simulink model "Distribution_v2"  (Simulink 7.9)
settings: Solver=VariableStepDiscrete  StartTime=0.0  StopTime=1000  RelTol=1e-3
libraries: simeventslib x35
(part 3 of 6)

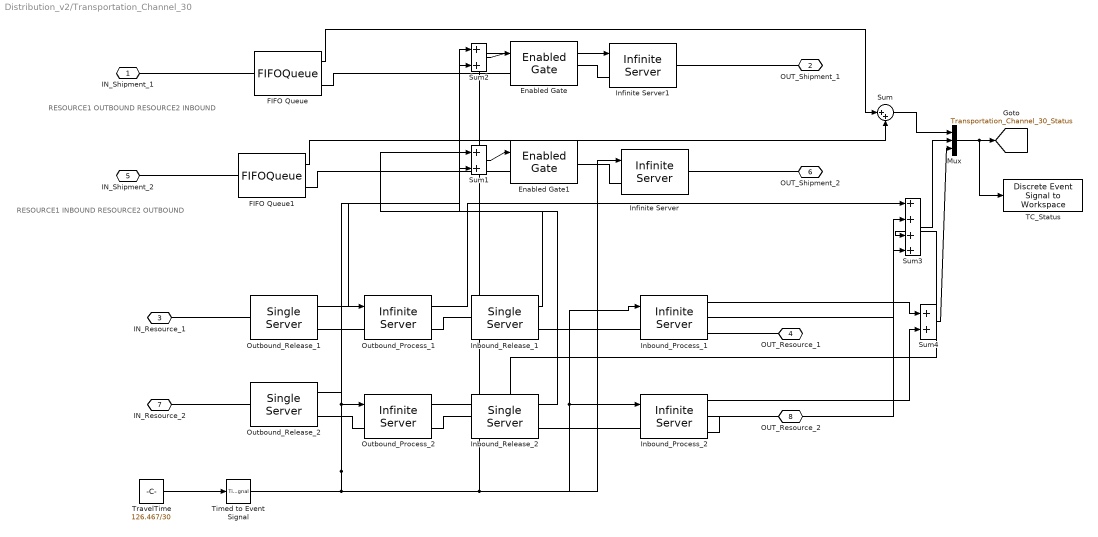
== system Distribution_v2/Transportation_Channel_30 ==
  note: RESOURCE1 OUTBOUND
      | RESOURCE2 INBOUND
  note: RESOURCE1 INBOUND
      | RESOURCE2 OUTBOUND
  Enabled Gate : EnabledGate
  Enabled Gate1 : EnabledGate
  FIFO Queue : FIFOQueue  Capacity=inf  StatNumberInBlock=on
      settings: OutputPortMap=o1
  FIFO Queue1 : FIFOQueue  Capacity=inf  StatNumberInBlock=on
      settings: OutputPortMap=o1
  Inbound_Process_1 : InfiniteServer  ServiceTimeFrom=Signal port t  ServiceTime=(76.7)/30  StatNumberDeparted=on  StatNumberInBlock=on
      settings: OutputPortMap=o0,o1
  Inbound_Process_2 : InfiniteServer  ServiceTimeFrom=Signal port t  ServiceTime=(76.7)/30  StatNumberDeparted=on  StatNumberInBlock=on
      settings: OutputPortMap=o0,o1
  Inbound_Release_1 : SingleServer  ServiceTime=0  StatNumberInBlock=on
      settings: OutputPortMap=o1
  Inbound_Release_2 : SingleServer  ServiceTime=0  StatNumberInBlock=on
      settings: OutputPortMap=o1
  Infinite Server : InfiniteServer  ServiceTimeFrom=Signal port t  ServiceTime=(76.7)/30
  Infinite Server1 : InfiniteServer  ServiceTimeFrom=Signal port t  ServiceTime=(76.7)/30
  Mux : Mux  Inputs=3
  Outbound_Process_1 : InfiniteServer  ServiceTimeFrom=Signal port t  ServiceTime=(76.7)/30  StatNumberInBlock=on
      settings: OutputPortMap=o1
  Outbound_Process_2 : InfiniteServer  ServiceTimeFrom=Signal port t  ServiceTime=(76.7)/30  StatNumberInBlock=on
      settings: OutputPortMap=o1
  Outbound_Release_1 : SingleServer  ServiceTime=0  StatNumberInBlock=on
      settings: OutputPortMap=o1
  Outbound_Release_2 : SingleServer  ServiceTime=0  StatNumberInBlock=on
      settings: OutputPortMap=o1
  Sum{,1..2,4} (4 alike) : Sum  Inputs=|++
  Sum3 : Sum  Inputs=|++++
  TC_Status : simeventslib/SimEvents Sinks/Discrete Event Signal to Workspace  VariableName=Transportation_Channel_30_Status  SaveFormat=Structure With Time  isMonitorOnly=off  isRecordIC=off
  Timed to Event Signal : TimedToEventSignal
  TravelTime : Constant  Value=126.467/30
  IN_Shipment_1 : PMIOPort  Port=1  Side=Left
  OUT_Shipment_1 : PMIOPort  Port=2  Side=Right
  IN_Resource_1 : PMIOPort  Port=3  Side=Left
  OUT_Resource_1 : PMIOPort  Port=4  Side=Right
  IN_Shipment_2 : PMIOPort  Port=5  Side=Left
  OUT_Shipment_2 : PMIOPort  Port=6  Side=Right
  IN_Resource_2 : PMIOPort  Port=7  Side=Left
  OUT_Resource_2 : PMIOPort  Port=8  Side=Right
  tag scope: Transportation_Channel_30_Status=global
  wires:
  Sum4/1 -> Mux/3
  Inbound_Process_2/1 -> Sum4/2
  Inbound_Process_1/1 -> Sum4/1
  Inbound_Process_2/2 -> Sum3/4
  Outbound_Process_2/1 -> Sum3/3
  Inbound_Process_1/2 -> Sum3/2
  Outbound_Process_1/1 -> Sum3/1
  Sum3/1 -> Mux/2
  Sum/1 -> Mux/1
  Mux/1 -> TC_Status/1, [Transportation_Channel_30_Status]
  Inbound_Release_2/1 -> Sum2/2
  Outbound_Release_1/1 -> Sum2/1
  Sum2/1 -> Enabled Gate/1
  Inbound_Release_1/1 -> Sum1/1
  Outbound_Release_2/1 -> Sum1/2
  Sum1/1 -> Enabled Gate1/1
  Timed to Event Signal/1 -> Infinite Server/1, Inbound_Process_2/1, Inbound_Process_1/1, Infinite Server1/1, Outbound_Process_2/1, Outbound_Process_1/1
  TravelTime/1 -> Timed to Event Signal/1
  FIFO Queue/1 -> Sum/1
  FIFO Queue1/1 -> Sum/2
  connections:
  Inbound_Process_1/RConn1 -- OUT_Resource_1/RConn1
  Outbound_Process_1/RConn1 -- Inbound_Release_1/LConn1
  Inbound_Release_1/RConn1 -- Inbound_Process_1/LConn1
  Outbound_Release_1/RConn1 -- Outbound_Process_1/LConn1
  Inbound_Process_2/RConn1 -- OUT_Resource_2/RConn1
  Inbound_Release_2/RConn1 -- Inbound_Process_2/LConn1
  Outbound_Process_2/RConn1 -- Inbound_Release_2/LConn1
  Outbound_Release_2/RConn1 -- Outbound_Process_2/LConn1
  IN_Resource_2/RConn1 -- Outbound_Release_2/LConn1
  Infinite Server1/RConn1 -- OUT_Shipment_1/RConn1
  Enabled Gate/RConn1 -- Infinite Server1/LConn1
  Infinite Server/LConn1 -- Enabled Gate1/RConn1
  OUT_Shipment_2/RConn1 -- Infinite Server/RConn1
  IN_Resource_1/RConn1 -- Outbound_Release_1/LConn1
  IN_Shipment_2/RConn1 -- FIFO Queue1/LConn1
  IN_Shipment_1/RConn1 -- FIFO Queue/LConn1
  Enabled Gate1/LConn1 -- FIFO Queue1/RConn1
  FIFO Queue/RConn1 -- Enabled Gate/LConn1

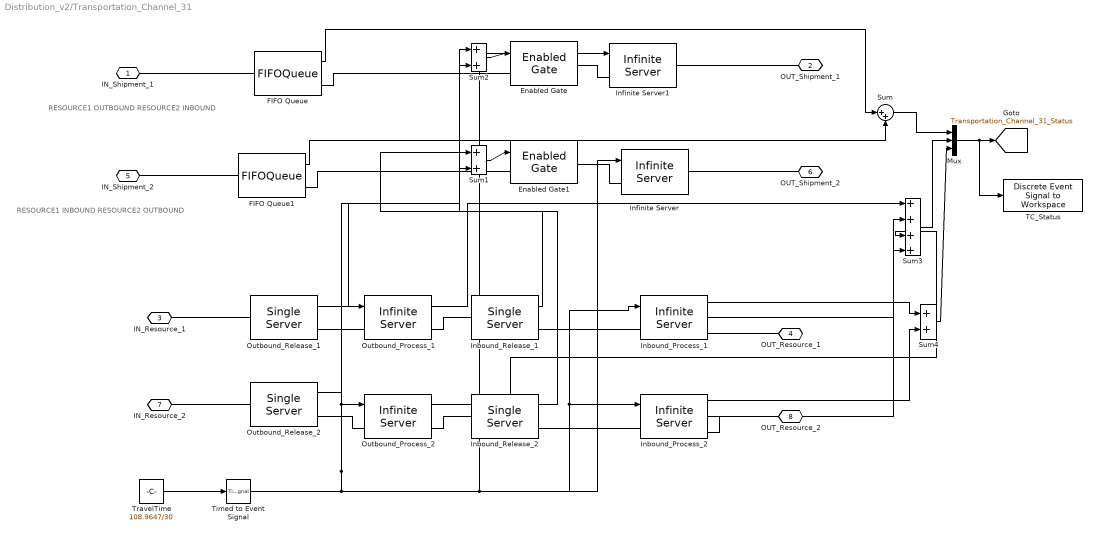
== system Distribution_v2/Transportation_Channel_31 ==
  note: RESOURCE1 OUTBOUND
      | RESOURCE2 INBOUND
  note: RESOURCE1 INBOUND
      | RESOURCE2 OUTBOUND
  Enabled Gate : EnabledGate
  Enabled Gate1 : EnabledGate
  FIFO Queue : FIFOQueue  Capacity=inf  StatNumberInBlock=on
      settings: OutputPortMap=o1
  FIFO Queue1 : FIFOQueue  Capacity=inf  StatNumberInBlock=on
      settings: OutputPortMap=o1
  Inbound_Process_1 : InfiniteServer  ServiceTimeFrom=Signal port t  ServiceTime=(76.7)/30  StatNumberDeparted=on  StatNumberInBlock=on
      settings: OutputPortMap=o0,o1
  Inbound_Process_2 : InfiniteServer  ServiceTimeFrom=Signal port t  ServiceTime=(76.7)/30  StatNumberDeparted=on  StatNumberInBlock=on
      settings: OutputPortMap=o0,o1
  Inbound_Release_1 : SingleServer  ServiceTime=0  StatNumberInBlock=on
      settings: OutputPortMap=o1
  Inbound_Release_2 : SingleServer  ServiceTime=0  StatNumberInBlock=on
      settings: OutputPortMap=o1
  Infinite Server : InfiniteServer  ServiceTimeFrom=Signal port t  ServiceTime=(76.7)/30
  Infinite Server1 : InfiniteServer  ServiceTimeFrom=Signal port t  ServiceTime=(76.7)/30
  Mux : Mux  Inputs=3
  Outbound_Process_1 : InfiniteServer  ServiceTimeFrom=Signal port t  ServiceTime=(76.7)/30  StatNumberInBlock=on
      settings: OutputPortMap=o1
  Outbound_Process_2 : InfiniteServer  ServiceTimeFrom=Signal port t  ServiceTime=(76.7)/30  StatNumberInBlock=on
      settings: OutputPortMap=o1
  Outbound_Release_1 : SingleServer  ServiceTime=0  StatNumberInBlock=on
      settings: OutputPortMap=o1
  Outbound_Release_2 : SingleServer  ServiceTime=0  StatNumberInBlock=on
      settings: OutputPortMap=o1
  Sum{,1..2,4} (4 alike) : Sum  Inputs=|++
  Sum3 : Sum  Inputs=|++++
  TC_Status : simeventslib/SimEvents Sinks/Discrete Event Signal to Workspace  VariableName=Transportation_Channel_31_Status  SaveFormat=Structure With Time  isMonitorOnly=off  isRecordIC=off
  Timed to Event Signal : TimedToEventSignal
  TravelTime : Constant  Value=108.9647/30
  IN_Shipment_1 : PMIOPort  Port=1  Side=Left
  OUT_Shipment_1 : PMIOPort  Port=2  Side=Right
  IN_Resource_1 : PMIOPort  Port=3  Side=Left
  OUT_Resource_1 : PMIOPort  Port=4  Side=Right
  IN_Shipment_2 : PMIOPort  Port=5  Side=Left
  OUT_Shipment_2 : PMIOPort  Port=6  Side=Right
  IN_Resource_2 : PMIOPort  Port=7  Side=Left
  OUT_Resource_2 : PMIOPort  Port=8  Side=Right
  tag scope: Transportation_Channel_31_Status=global
  wires:
  Sum4/1 -> Mux/3
  Inbound_Process_2/1 -> Sum4/2
  Inbound_Process_1/1 -> Sum4/1
  Inbound_Process_2/2 -> Sum3/4
  Outbound_Process_2/1 -> Sum3/3
  Inbound_Process_1/2 -> Sum3/2
  Outbound_Process_1/1 -> Sum3/1
  Sum3/1 -> Mux/2
  Sum/1 -> Mux/1
  Mux/1 -> TC_Status/1, [Transportation_Channel_31_Status]
  Inbound_Release_2/1 -> Sum2/2
  Outbound_Release_1/1 -> Sum2/1
  Sum2/1 -> Enabled Gate/1
  Inbound_Release_1/1 -> Sum1/1
  Outbound_Release_2/1 -> Sum1/2
  Sum1/1 -> Enabled Gate1/1
  Timed to Event Signal/1 -> Infinite Server/1, Inbound_Process_2/1, Inbound_Process_1/1, Infinite Server1/1, Outbound_Process_2/1, Outbound_Process_1/1
  TravelTime/1 -> Timed to Event Signal/1
  FIFO Queue/1 -> Sum/1
  FIFO Queue1/1 -> Sum/2
  connections:
  Inbound_Process_1/RConn1 -- OUT_Resource_1/RConn1
  Outbound_Process_1/RConn1 -- Inbound_Release_1/LConn1
  Inbound_Release_1/RConn1 -- Inbound_Process_1/LConn1
  Outbound_Release_1/RConn1 -- Outbound_Process_1/LConn1
  Inbound_Process_2/RConn1 -- OUT_Resource_2/RConn1
  Inbound_Release_2/RConn1 -- Inbound_Process_2/LConn1
  Outbound_Process_2/RConn1 -- Inbound_Release_2/LConn1
  Outbound_Release_2/RConn1 -- Outbound_Process_2/LConn1
  IN_Resource_2/RConn1 -- Outbound_Release_2/LConn1
  Infinite Server1/RConn1 -- OUT_Shipment_1/RConn1
  Enabled Gate/RConn1 -- Infinite Server1/LConn1
  Infinite Server/LConn1 -- Enabled Gate1/RConn1
  OUT_Shipment_2/RConn1 -- Infinite Server/RConn1
  IN_Resource_1/RConn1 -- Outbound_Release_1/LConn1
  IN_Shipment_2/RConn1 -- FIFO Queue1/LConn1
  IN_Shipment_1/RConn1 -- FIFO Queue/LConn1
  Enabled Gate1/LConn1 -- FIFO Queue1/RConn1
  FIFO Queue/RConn1 -- Enabled Gate/LConn1

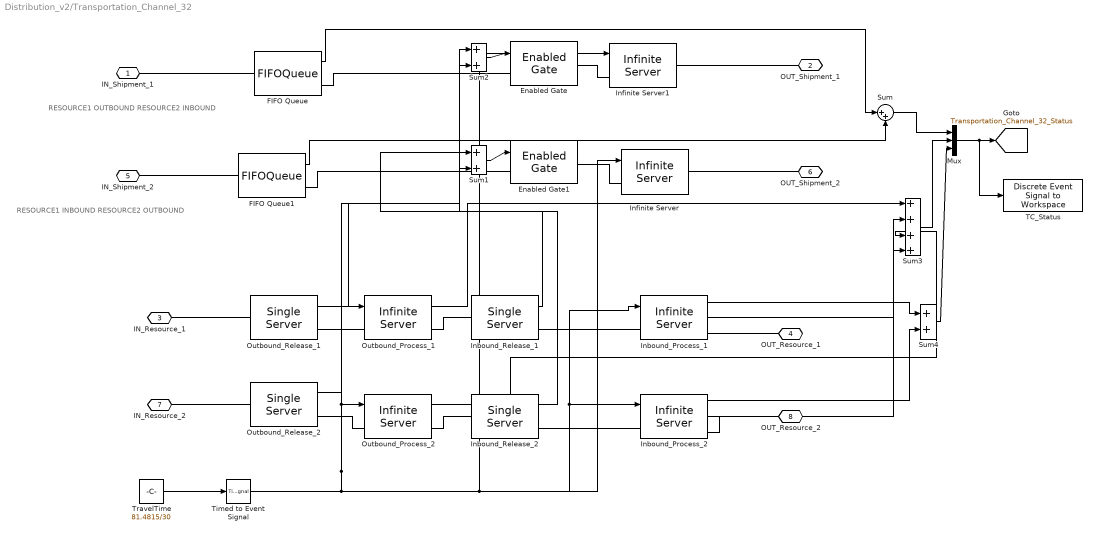
== system Distribution_v2/Transportation_Channel_32 ==
  note: RESOURCE1 OUTBOUND
      | RESOURCE2 INBOUND
  note: RESOURCE1 INBOUND
      | RESOURCE2 OUTBOUND
  Enabled Gate : EnabledGate
  Enabled Gate1 : EnabledGate
  FIFO Queue : FIFOQueue  Capacity=inf  StatNumberInBlock=on
      settings: OutputPortMap=o1
  FIFO Queue1 : FIFOQueue  Capacity=inf  StatNumberInBlock=on
      settings: OutputPortMap=o1
  Inbound_Process_1 : InfiniteServer  ServiceTimeFrom=Signal port t  ServiceTime=(76.7)/30  StatNumberDeparted=on  StatNumberInBlock=on
      settings: OutputPortMap=o0,o1
  Inbound_Process_2 : InfiniteServer  ServiceTimeFrom=Signal port t  ServiceTime=(76.7)/30  StatNumberDeparted=on  StatNumberInBlock=on
      settings: OutputPortMap=o0,o1
  Inbound_Release_1 : SingleServer  ServiceTime=0  StatNumberInBlock=on
      settings: OutputPortMap=o1
  Inbound_Release_2 : SingleServer  ServiceTime=0  StatNumberInBlock=on
      settings: OutputPortMap=o1
  Infinite Server : InfiniteServer  ServiceTimeFrom=Signal port t  ServiceTime=(76.7)/30
  Infinite Server1 : InfiniteServer  ServiceTimeFrom=Signal port t  ServiceTime=(76.7)/30
  Mux : Mux  Inputs=3
  Outbound_Process_1 : InfiniteServer  ServiceTimeFrom=Signal port t  ServiceTime=(76.7)/30  StatNumberInBlock=on
      settings: OutputPortMap=o1
  Outbound_Process_2 : InfiniteServer  ServiceTimeFrom=Signal port t  ServiceTime=(76.7)/30  StatNumberInBlock=on
      settings: OutputPortMap=o1
  Outbound_Release_1 : SingleServer  ServiceTime=0  StatNumberInBlock=on
      settings: OutputPortMap=o1
  Outbound_Release_2 : SingleServer  ServiceTime=0  StatNumberInBlock=on
      settings: OutputPortMap=o1
  Sum{,1..2,4} (4 alike) : Sum  Inputs=|++
  Sum3 : Sum  Inputs=|++++
  TC_Status : simeventslib/SimEvents Sinks/Discrete Event Signal to Workspace  VariableName=Transportation_Channel_32_Status  SaveFormat=Structure With Time  isMonitorOnly=off  isRecordIC=off
  Timed to Event Signal : TimedToEventSignal
  TravelTime : Constant  Value=81.4815/30
  IN_Shipment_1 : PMIOPort  Port=1  Side=Left
  OUT_Shipment_1 : PMIOPort  Port=2  Side=Right
  IN_Resource_1 : PMIOPort  Port=3  Side=Left
  OUT_Resource_1 : PMIOPort  Port=4  Side=Right
  IN_Shipment_2 : PMIOPort  Port=5  Side=Left
  OUT_Shipment_2 : PMIOPort  Port=6  Side=Right
  IN_Resource_2 : PMIOPort  Port=7  Side=Left
  OUT_Resource_2 : PMIOPort  Port=8  Side=Right
  tag scope: Transportation_Channel_32_Status=global
  wires:
  Sum4/1 -> Mux/3
  Inbound_Process_2/1 -> Sum4/2
  Inbound_Process_1/1 -> Sum4/1
  Inbound_Process_2/2 -> Sum3/4
  Outbound_Process_2/1 -> Sum3/3
  Inbound_Process_1/2 -> Sum3/2
  Outbound_Process_1/1 -> Sum3/1
  Sum3/1 -> Mux/2
  Sum/1 -> Mux/1
  Mux/1 -> TC_Status/1, [Transportation_Channel_32_Status]
  Inbound_Release_2/1 -> Sum2/2
  Outbound_Release_1/1 -> Sum2/1
  Sum2/1 -> Enabled Gate/1
  Inbound_Release_1/1 -> Sum1/1
  Outbound_Release_2/1 -> Sum1/2
  Sum1/1 -> Enabled Gate1/1
  Timed to Event Signal/1 -> Infinite Server/1, Inbound_Process_2/1, Inbound_Process_1/1, Infinite Server1/1, Outbound_Process_2/1, Outbound_Process_1/1
  TravelTime/1 -> Timed to Event Signal/1
  FIFO Queue/1 -> Sum/1
  FIFO Queue1/1 -> Sum/2
  connections:
  Inbound_Process_1/RConn1 -- OUT_Resource_1/RConn1
  Outbound_Process_1/RConn1 -- Inbound_Release_1/LConn1
  Inbound_Release_1/RConn1 -- Inbound_Process_1/LConn1
  Outbound_Release_1/RConn1 -- Outbound_Process_1/LConn1
  Inbound_Process_2/RConn1 -- OUT_Resource_2/RConn1
  Inbound_Release_2/RConn1 -- Inbound_Process_2/LConn1
  Outbound_Process_2/RConn1 -- Inbound_Release_2/LConn1
  Outbound_Release_2/RConn1 -- Outbound_Process_2/LConn1
  IN_Resource_2/RConn1 -- Outbound_Release_2/LConn1
  Infinite Server1/RConn1 -- OUT_Shipment_1/RConn1
  Enabled Gate/RConn1 -- Infinite Server1/LConn1
  Infinite Server/LConn1 -- Enabled Gate1/RConn1
  OUT_Shipment_2/RConn1 -- Infinite Server/RConn1
  IN_Resource_1/RConn1 -- Outbound_Release_1/LConn1
  IN_Shipment_2/RConn1 -- FIFO Queue1/LConn1
  IN_Shipment_1/RConn1 -- FIFO Queue/LConn1
  Enabled Gate1/LConn1 -- FIFO Queue1/RConn1
  FIFO Queue/RConn1 -- Enabled Gate/LConn1

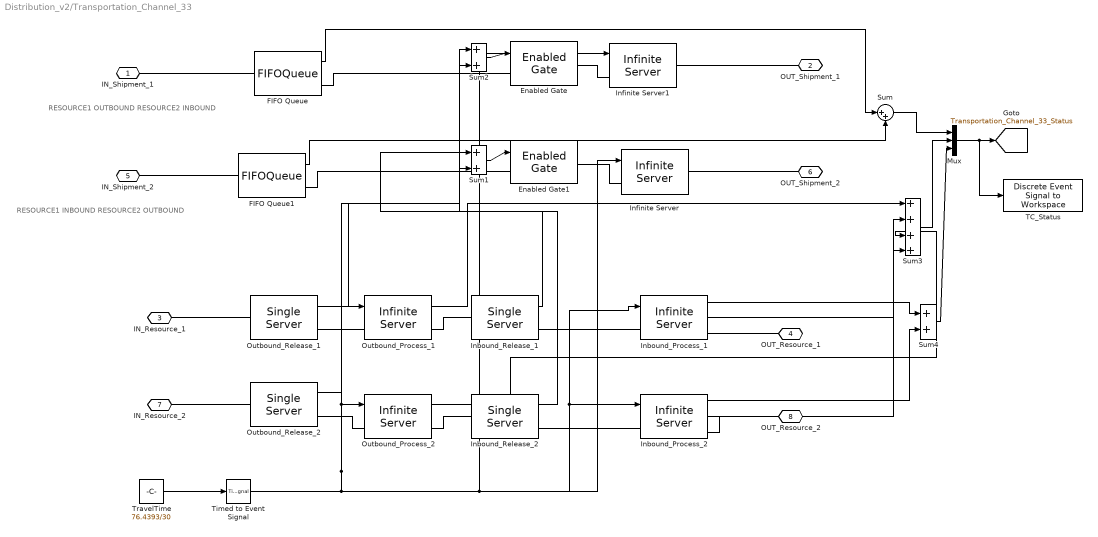
== system Distribution_v2/Transportation_Channel_33 ==
  note: RESOURCE1 OUTBOUND
      | RESOURCE2 INBOUND
  note: RESOURCE1 INBOUND
      | RESOURCE2 OUTBOUND
  Enabled Gate : EnabledGate
  Enabled Gate1 : EnabledGate
  FIFO Queue : FIFOQueue  Capacity=inf  StatNumberInBlock=on
      settings: OutputPortMap=o1
  FIFO Queue1 : FIFOQueue  Capacity=inf  StatNumberInBlock=on
      settings: OutputPortMap=o1
  Inbound_Process_1 : InfiniteServer  ServiceTimeFrom=Signal port t  ServiceTime=(76.7)/30  StatNumberDeparted=on  StatNumberInBlock=on
      settings: OutputPortMap=o0,o1
  Inbound_Process_2 : InfiniteServer  ServiceTimeFrom=Signal port t  ServiceTime=(76.7)/30  StatNumberDeparted=on  StatNumberInBlock=on
      settings: OutputPortMap=o0,o1
  Inbound_Release_1 : SingleServer  ServiceTime=0  StatNumberInBlock=on
      settings: OutputPortMap=o1
  Inbound_Release_2 : SingleServer  ServiceTime=0  StatNumberInBlock=on
      settings: OutputPortMap=o1
  Infinite Server : InfiniteServer  ServiceTimeFrom=Signal port t  ServiceTime=(76.7)/30
  Infinite Server1 : InfiniteServer  ServiceTimeFrom=Signal port t  ServiceTime=(76.7)/30
  Mux : Mux  Inputs=3
  Outbound_Process_1 : InfiniteServer  ServiceTimeFrom=Signal port t  ServiceTime=(76.7)/30  StatNumberInBlock=on
      settings: OutputPortMap=o1
  Outbound_Process_2 : InfiniteServer  ServiceTimeFrom=Signal port t  ServiceTime=(76.7)/30  StatNumberInBlock=on
      settings: OutputPortMap=o1
  Outbound_Release_1 : SingleServer  ServiceTime=0  StatNumberInBlock=on
      settings: OutputPortMap=o1
  Outbound_Release_2 : SingleServer  ServiceTime=0  StatNumberInBlock=on
      settings: OutputPortMap=o1
  Sum{,1..2,4} (4 alike) : Sum  Inputs=|++
  Sum3 : Sum  Inputs=|++++
  TC_Status : simeventslib/SimEvents Sinks/Discrete Event Signal to Workspace  VariableName=Transportation_Channel_33_Status  SaveFormat=Structure With Time  isMonitorOnly=off  isRecordIC=off
  Timed to Event Signal : TimedToEventSignal
  TravelTime : Constant  Value=76.4393/30
  IN_Shipment_1 : PMIOPort  Port=1  Side=Left
  OUT_Shipment_1 : PMIOPort  Port=2  Side=Right
  IN_Resource_1 : PMIOPort  Port=3  Side=Left
  OUT_Resource_1 : PMIOPort  Port=4  Side=Right
  IN_Shipment_2 : PMIOPort  Port=5  Side=Left
  OUT_Shipment_2 : PMIOPort  Port=6  Side=Right
  IN_Resource_2 : PMIOPort  Port=7  Side=Left
  OUT_Resource_2 : PMIOPort  Port=8  Side=Right
  tag scope: Transportation_Channel_33_Status=global
  wires:
  Sum4/1 -> Mux/3
  Inbound_Process_2/1 -> Sum4/2
  Inbound_Process_1/1 -> Sum4/1
  Inbound_Process_2/2 -> Sum3/4
  Outbound_Process_2/1 -> Sum3/3
  Inbound_Process_1/2 -> Sum3/2
  Outbound_Process_1/1 -> Sum3/1
  Sum3/1 -> Mux/2
  Sum/1 -> Mux/1
  Mux/1 -> TC_Status/1, [Transportation_Channel_33_Status]
  Inbound_Release_2/1 -> Sum2/2
  Outbound_Release_1/1 -> Sum2/1
  Sum2/1 -> Enabled Gate/1
  Inbound_Release_1/1 -> Sum1/1
  Outbound_Release_2/1 -> Sum1/2
  Sum1/1 -> Enabled Gate1/1
  Timed to Event Signal/1 -> Infinite Server/1, Inbound_Process_2/1, Inbound_Process_1/1, Infinite Server1/1, Outbound_Process_2/1, Outbound_Process_1/1
  TravelTime/1 -> Timed to Event Signal/1
  FIFO Queue/1 -> Sum/1
  FIFO Queue1/1 -> Sum/2
  connections:
  Inbound_Process_1/RConn1 -- OUT_Resource_1/RConn1
  Outbound_Process_1/RConn1 -- Inbound_Release_1/LConn1
  Inbound_Release_1/RConn1 -- Inbound_Process_1/LConn1
  Outbound_Release_1/RConn1 -- Outbound_Process_1/LConn1
  Inbound_Process_2/RConn1 -- OUT_Resource_2/RConn1
  Inbound_Release_2/RConn1 -- Inbound_Process_2/LConn1
  Outbound_Process_2/RConn1 -- Inbound_Release_2/LConn1
  Outbound_Release_2/RConn1 -- Outbound_Process_2/LConn1
  IN_Resource_2/RConn1 -- Outbound_Release_2/LConn1
  Infinite Server1/RConn1 -- OUT_Shipment_1/RConn1
  Enabled Gate/RConn1 -- Infinite Server1/LConn1
  Infinite Server/LConn1 -- Enabled Gate1/RConn1
  OUT_Shipment_2/RConn1 -- Infinite Server/RConn1
  IN_Resource_1/RConn1 -- Outbound_Release_1/LConn1
  IN_Shipment_2/RConn1 -- FIFO Queue1/LConn1
  IN_Shipment_1/RConn1 -- FIFO Queue/LConn1
  Enabled Gate1/LConn1 -- FIFO Queue1/RConn1
  FIFO Queue/RConn1 -- Enabled Gate/LConn1

== system Distribution_v2/Transportation_Channel_34 ==
  note: RESOURCE1 OUTBOUND
      | RESOURCE2 INBOUND
  note: RESOURCE1 INBOUND
      | RESOURCE2 OUTBOUND
  Enabled Gate : EnabledGate
  Enabled Gate1 : EnabledGate
  FIFO Queue : FIFOQueue  Capacity=inf  StatNumberInBlock=on
      settings: OutputPortMap=o1
  FIFO Queue1 : FIFOQueue  Capacity=inf  StatNumberInBlock=on
      settings: OutputPortMap=o1
  Inbound_Process_1 : InfiniteServer  ServiceTimeFrom=Signal port t  ServiceTime=(76.7)/30  StatNumberDeparted=on  StatNumberInBlock=on
      settings: OutputPortMap=o0,o1
  Inbound_Process_2 : InfiniteServer  ServiceTimeFrom=Signal port t  ServiceTime=(76.7)/30  StatNumberDeparted=on  StatNumberInBlock=on
      settings: OutputPortMap=o0,o1
  Inbound_Release_1 : SingleServer  ServiceTime=0  StatNumberInBlock=on
      settings: OutputPortMap=o1
  Inbound_Release_2 : SingleServer  ServiceTime=0  StatNumberInBlock=on
      settings: OutputPortMap=o1
  Infinite Server : InfiniteServer  ServiceTimeFrom=Signal port t  ServiceTime=(76.7)/30
  Infinite Server1 : InfiniteServer  ServiceTimeFrom=Signal port t  ServiceTime=(76.7)/30
  Mux : Mux  Inputs=3
  Outbound_Process_1 : InfiniteServer  ServiceTimeFrom=Signal port t  ServiceTime=(76.7)/30  StatNumberInBlock=on
      settings: OutputPortMap=o1
  Outbound_Process_2 : InfiniteServer  ServiceTimeFrom=Signal port t  ServiceTime=(76.7)/30  StatNumberInBlock=on
      settings: OutputPortMap=o1
  Outbound_Release_1 : SingleServer  ServiceTime=0  StatNumberInBlock=on
      settings: OutputPortMap=o1
  Outbound_Release_2 : SingleServer  ServiceTime=0  StatNumberInBlock=on
      settings: OutputPortMap=o1
  Sum{,1..2,4} (4 alike) : Sum  Inputs=|++
  Sum3 : Sum  Inputs=|++++
  TC_Status : simeventslib/SimEvents Sinks/Discrete Event Signal to Workspace  VariableName=Transportation_Channel_34_Status  SaveFormat=Structure With Time  isMonitorOnly=off  isRecordIC=off
  Timed to Event Signal : TimedToEventSignal
  TravelTime : Constant  Value=35.0759/30
  IN_Shipment_1 : PMIOPort  Port=1  Side=Left
  OUT_Shipment_1 : PMIOPort  Port=2  Side=Right
  IN_Resource_1 : PMIOPort  Port=3  Side=Left
  OUT_Resource_1 : PMIOPort  Port=4  Side=Right
  IN_Shipment_2 : PMIOPort  Port=5  Side=Left
  OUT_Shipment_2 : PMIOPort  Port=6  Side=Right
  IN_Resource_2 : PMIOPort  Port=7  Side=Left
  OUT_Resource_2 : PMIOPort  Port=8  Side=Right
  tag scope: Transportation_Channel_34_Status=global
  wires:
  Sum4/1 -> Mux/3
  Inbound_Process_2/1 -> Sum4/2
  Inbound_Process_1/1 -> Sum4/1
  Inbound_Process_2/2 -> Sum3/4
  Outbound_Process_2/1 -> Sum3/3
  Inbound_Process_1/2 -> Sum3/2
  Outbound_Process_1/1 -> Sum3/1
  Sum3/1 -> Mux/2
  Sum/1 -> Mux/1
  Mux/1 -> TC_Status/1, [Transportation_Channel_34_Status]
  Inbound_Release_2/1 -> Sum2/2
  Outbound_Release_1/1 -> Sum2/1
  Sum2/1 -> Enabled Gate/1
  Inbound_Release_1/1 -> Sum1/1
  Outbound_Release_2/1 -> Sum1/2
  Sum1/1 -> Enabled Gate1/1
  Timed to Event Signal/1 -> Infinite Server/1, Inbound_Process_2/1, Inbound_Process_1/1, Infinite Server1/1, Outbound_Process_2/1, Outbound_Process_1/1
  TravelTime/1 -> Timed to Event Signal/1
  FIFO Queue/1 -> Sum/1
  FIFO Queue1/1 -> Sum/2
  connections:
  Inbound_Process_1/RConn1 -- OUT_Resource_1/RConn1
  Outbound_Process_1/RConn1 -- Inbound_Release_1/LConn1
  Inbound_Release_1/RConn1 -- Inbound_Process_1/LConn1
  Outbound_Release_1/RConn1 -- Outbound_Process_1/LConn1
  Inbound_Process_2/RConn1 -- OUT_Resource_2/RConn1
  Inbound_Release_2/RConn1 -- Inbound_Process_2/LConn1
  Outbound_Process_2/RConn1 -- Inbound_Release_2/LConn1
  Outbound_Release_2/RConn1 -- Outbound_Process_2/LConn1
  IN_Resource_2/RConn1 -- Outbound_Release_2/LConn1
  Infinite Server1/RConn1 -- OUT_Shipment_1/RConn1
  Enabled Gate/RConn1 -- Infinite Server1/LConn1
  Infinite Server/LConn1 -- Enabled Gate1/RConn1
  OUT_Shipment_2/RConn1 -- Infinite Server/RConn1
  IN_Resource_1/RConn1 -- Outbound_Release_1/LConn1
  IN_Shipment_2/RConn1 -- FIFO Queue1/LConn1
  IN_Shipment_1/RConn1 -- FIFO Queue/LConn1
  Enabled Gate1/LConn1 -- FIFO Queue1/RConn1
  FIFO Queue/RConn1 -- Enabled Gate/LConn1

== system Distribution_v2/Transportation_Channel_35 ==
  note: RESOURCE1 OUTBOUND
      | RESOURCE2 INBOUND
  note: RESOURCE1 INBOUND
      | RESOURCE2 OUTBOUND
  Enabled Gate : EnabledGate
  Enabled Gate1 : EnabledGate
  FIFO Queue : FIFOQueue  Capacity=inf  StatNumberInBlock=on
      settings: OutputPortMap=o1
  FIFO Queue1 : FIFOQueue  Capacity=inf  StatNumberInBlock=on
      settings: OutputPortMap=o1
  Inbound_Process_1 : InfiniteServer  ServiceTimeFrom=Signal port t  ServiceTime=(76.7)/30  StatNumberDeparted=on  StatNumberInBlock=on
      settings: OutputPortMap=o0,o1
  Inbound_Process_2 : InfiniteServer  ServiceTimeFrom=Signal port t  ServiceTime=(76.7)/30  StatNumberDeparted=on  StatNumberInBlock=on
      settings: OutputPortMap=o0,o1
  Inbound_Release_1 : SingleServer  ServiceTime=0  StatNumberInBlock=on
      settings: OutputPortMap=o1
  Inbound_Release_2 : SingleServer  ServiceTime=0  StatNumberInBlock=on
      settings: OutputPortMap=o1
  Infinite Server : InfiniteServer  ServiceTimeFrom=Signal port t  ServiceTime=(76.7)/30
  Infinite Server1 : InfiniteServer  ServiceTimeFrom=Signal port t  ServiceTime=(76.7)/30
  Mux : Mux  Inputs=3
  Outbound_Process_1 : InfiniteServer  ServiceTimeFrom=Signal port t  ServiceTime=(76.7)/30  StatNumberInBlock=on
      settings: OutputPortMap=o1
  Outbound_Process_2 : InfiniteServer  ServiceTimeFrom=Signal port t  ServiceTime=(76.7)/30  StatNumberInBlock=on
      settings: OutputPortMap=o1
  Outbound_Release_1 : SingleServer  ServiceTime=0  StatNumberInBlock=on
      settings: OutputPortMap=o1
  Outbound_Release_2 : SingleServer  ServiceTime=0  StatNumberInBlock=on
      settings: OutputPortMap=o1
  Sum{,1..2,4} (4 alike) : Sum  Inputs=|++
  Sum3 : Sum  Inputs=|++++
  TC_Status : simeventslib/SimEvents Sinks/Discrete Event Signal to Workspace  VariableName=Transportation_Channel_35_Status  SaveFormat=Structure With Time  isMonitorOnly=off  isRecordIC=off
  Timed to Event Signal : TimedToEventSignal
  TravelTime : Constant  Value=67.7533/30
  IN_Shipment_1 : PMIOPort  Port=1  Side=Left
  OUT_Shipment_1 : PMIOPort  Port=2  Side=Right
  IN_Resource_1 : PMIOPort  Port=3  Side=Left
  OUT_Resource_1 : PMIOPort  Port=4  Side=Right
  IN_Shipment_2 : PMIOPort  Port=5  Side=Left
  OUT_Shipment_2 : PMIOPort  Port=6  Side=Right
  IN_Resource_2 : PMIOPort  Port=7  Side=Left
  OUT_Resource_2 : PMIOPort  Port=8  Side=Right
  tag scope: Transportation_Channel_35_Status=global
  wires:
  Sum4/1 -> Mux/3
  Inbound_Process_2/1 -> Sum4/2
  Inbound_Process_1/1 -> Sum4/1
  Inbound_Process_2/2 -> Sum3/4
  Outbound_Process_2/1 -> Sum3/3
  Inbound_Process_1/2 -> Sum3/2
  Outbound_Process_1/1 -> Sum3/1
  Sum3/1 -> Mux/2
  Sum/1 -> Mux/1
  Mux/1 -> TC_Status/1, [Transportation_Channel_35_Status]
  Inbound_Release_2/1 -> Sum2/2
  Outbound_Release_1/1 -> Sum2/1
  Sum2/1 -> Enabled Gate/1
  Inbound_Release_1/1 -> Sum1/1
  Outbound_Release_2/1 -> Sum1/2
  Sum1/1 -> Enabled Gate1/1
  Timed to Event Signal/1 -> Infinite Server/1, Inbound_Process_2/1, Inbound_Process_1/1, Infinite Server1/1, Outbound_Process_2/1, Outbound_Process_1/1
  TravelTime/1 -> Timed to Event Signal/1
  FIFO Queue/1 -> Sum/1
  FIFO Queue1/1 -> Sum/2
  connections:
  Inbound_Process_1/RConn1 -- OUT_Resource_1/RConn1
  Outbound_Process_1/RConn1 -- Inbound_Release_1/LConn1
  Inbound_Release_1/RConn1 -- Inbound_Process_1/LConn1
  Outbound_Release_1/RConn1 -- Outbound_Process_1/LConn1
  Inbound_Process_2/RConn1 -- OUT_Resource_2/RConn1
  Inbound_Release_2/RConn1 -- Inbound_Process_2/LConn1
  Outbound_Process_2/RConn1 -- Inbound_Release_2/LConn1
  Outbound_Release_2/RConn1 -- Outbound_Process_2/LConn1
  IN_Resource_2/RConn1 -- Outbound_Release_2/LConn1
  Infinite Server1/RConn1 -- OUT_Shipment_1/RConn1
  Enabled Gate/RConn1 -- Infinite Server1/LConn1
  Infinite Server/LConn1 -- Enabled Gate1/RConn1
  OUT_Shipment_2/RConn1 -- Infinite Server/RConn1
  IN_Resource_1/RConn1 -- Outbound_Release_1/LConn1
  IN_Shipment_2/RConn1 -- FIFO Queue1/LConn1
  IN_Shipment_1/RConn1 -- FIFO Queue/LConn1
  Enabled Gate1/LConn1 -- FIFO Queue1/RConn1
  FIFO Queue/RConn1 -- Enabled Gate/LConn1

== system Distribution_v2/Transportation_Channel_36 ==
  note: RESOURCE1 OUTBOUND
      | RESOURCE2 INBOUND
  note: RESOURCE1 INBOUND
      | RESOURCE2 OUTBOUND
  Enabled Gate : EnabledGate
  Enabled Gate1 : EnabledGate
  FIFO Queue : FIFOQueue  Capacity=inf  StatNumberInBlock=on
      settings: OutputPortMap=o1
  FIFO Queue1 : FIFOQueue  Capacity=inf  StatNumberInBlock=on
      settings: OutputPortMap=o1
  Inbound_Process_1 : InfiniteServer  ServiceTimeFrom=Signal port t  ServiceTime=(76.7)/30  StatNumberDeparted=on  StatNumberInBlock=on
      settings: OutputPortMap=o0,o1
  Inbound_Process_2 : InfiniteServer  ServiceTimeFrom=Signal port t  ServiceTime=(76.7)/30  StatNumberDeparted=on  StatNumberInBlock=on
      settings: OutputPortMap=o0,o1
  Inbound_Release_1 : SingleServer  ServiceTime=0  StatNumberInBlock=on
      settings: OutputPortMap=o1
  Inbound_Release_2 : SingleServer  ServiceTime=0  StatNumberInBlock=on
      settings: OutputPortMap=o1
  Infinite Server : InfiniteServer  ServiceTimeFrom=Signal port t  ServiceTime=(76.7)/30
  Infinite Server1 : InfiniteServer  ServiceTimeFrom=Signal port t  ServiceTime=(76.7)/30
  Mux : Mux  Inputs=3
  Outbound_Process_1 : InfiniteServer  ServiceTimeFrom=Signal port t  ServiceTime=(76.7)/30  StatNumberInBlock=on
      settings: OutputPortMap=o1
  Outbound_Process_2 : InfiniteServer  ServiceTimeFrom=Signal port t  ServiceTime=(76.7)/30  StatNumberInBlock=on
      settings: OutputPortMap=o1
  Outbound_Release_1 : SingleServer  ServiceTime=0  StatNumberInBlock=on
      settings: OutputPortMap=o1
  Outbound_Release_2 : SingleServer  ServiceTime=0  StatNumberInBlock=on
      settings: OutputPortMap=o1
  Sum{,1..2,4} (4 alike) : Sum  Inputs=|++
  Sum3 : Sum  Inputs=|++++
  TC_Status : simeventslib/SimEvents Sinks/Discrete Event Signal to Workspace  VariableName=Transportation_Channel_36_Status  SaveFormat=Structure With Time  isMonitorOnly=off  isRecordIC=off
  Timed to Event Signal : TimedToEventSignal
  TravelTime : Constant  Value=84.0688/30
  IN_Shipment_1 : PMIOPort  Port=1  Side=Left
  OUT_Shipment_1 : PMIOPort  Port=2  Side=Right
  IN_Resource_1 : PMIOPort  Port=3  Side=Left
  OUT_Resource_1 : PMIOPort  Port=4  Side=Right
  IN_Shipment_2 : PMIOPort  Port=5  Side=Left
  OUT_Shipment_2 : PMIOPort  Port=6  Side=Right
  IN_Resource_2 : PMIOPort  Port=7  Side=Left
  OUT_Resource_2 : PMIOPort  Port=8  Side=Right
  tag scope: Transportation_Channel_36_Status=global
  wires:
  Sum4/1 -> Mux/3
  Inbound_Process_2/1 -> Sum4/2
  Inbound_Process_1/1 -> Sum4/1
  Inbound_Process_2/2 -> Sum3/4
  Outbound_Process_2/1 -> Sum3/3
  Inbound_Process_1/2 -> Sum3/2
  Outbound_Process_1/1 -> Sum3/1
  Sum3/1 -> Mux/2
  Sum/1 -> Mux/1
  Mux/1 -> TC_Status/1, [Transportation_Channel_36_Status]
  Inbound_Release_2/1 -> Sum2/2
  Outbound_Release_1/1 -> Sum2/1
  Sum2/1 -> Enabled Gate/1
  Inbound_Release_1/1 -> Sum1/1
  Outbound_Release_2/1 -> Sum1/2
  Sum1/1 -> Enabled Gate1/1
  Timed to Event Signal/1 -> Infinite Server/1, Inbound_Process_2/1, Inbound_Process_1/1, Infinite Server1/1, Outbound_Process_2/1, Outbound_Process_1/1
  TravelTime/1 -> Timed to Event Signal/1
  FIFO Queue/1 -> Sum/1
  FIFO Queue1/1 -> Sum/2
  connections:
  Inbound_Process_1/RConn1 -- OUT_Resource_1/RConn1
  Outbound_Process_1/RConn1 -- Inbound_Release_1/LConn1
  Inbound_Release_1/RConn1 -- Inbound_Process_1/LConn1
  Outbound_Release_1/RConn1 -- Outbound_Process_1/LConn1
  Inbound_Process_2/RConn1 -- OUT_Resource_2/RConn1
  Inbound_Release_2/RConn1 -- Inbound_Process_2/LConn1
  Outbound_Process_2/RConn1 -- Inbound_Release_2/LConn1
  Outbound_Release_2/RConn1 -- Outbound_Process_2/LConn1
  IN_Resource_2/RConn1 -- Outbound_Release_2/LConn1
  Infinite Server1/RConn1 -- OUT_Shipment_1/RConn1
  Enabled Gate/RConn1 -- Infinite Server1/LConn1
  Infinite Server/LConn1 -- Enabled Gate1/RConn1
  OUT_Shipment_2/RConn1 -- Infinite Server/RConn1
  IN_Resource_1/RConn1 -- Outbound_Release_1/LConn1
  IN_Shipment_2/RConn1 -- FIFO Queue1/LConn1
  IN_Shipment_1/RConn1 -- FIFO Queue/LConn1
  Enabled Gate1/LConn1 -- FIFO Queue1/RConn1
  FIFO Queue/RConn1 -- Enabled Gate/LConn1

== system Distribution_v2/Transportation_Channel_37 ==
  note: RESOURCE1 OUTBOUND
      | RESOURCE2 INBOUND
  note: RESOURCE1 INBOUND
      | RESOURCE2 OUTBOUND
  Enabled Gate : EnabledGate
  Enabled Gate1 : EnabledGate
  FIFO Queue : FIFOQueue  Capacity=inf  StatNumberInBlock=on
      settings: OutputPortMap=o1
  FIFO Queue1 : FIFOQueue  Capacity=inf  StatNumberInBlock=on
      settings: OutputPortMap=o1
  Inbound_Process_1 : InfiniteServer  ServiceTimeFrom=Signal port t  ServiceTime=(76.7)/30  StatNumberDeparted=on  StatNumberInBlock=on
      settings: OutputPortMap=o0,o1
  Inbound_Process_2 : InfiniteServer  ServiceTimeFrom=Signal port t  ServiceTime=(76.7)/30  StatNumberDeparted=on  StatNumberInBlock=on
      settings: OutputPortMap=o0,o1
  Inbound_Release_1 : SingleServer  ServiceTime=0  StatNumberInBlock=on
      settings: OutputPortMap=o1
  Inbound_Release_2 : SingleServer  ServiceTime=0  StatNumberInBlock=on
      settings: OutputPortMap=o1
  Infinite Server : InfiniteServer  ServiceTimeFrom=Signal port t  ServiceTime=(76.7)/30
  Infinite Server1 : InfiniteServer  ServiceTimeFrom=Signal port t  ServiceTime=(76.7)/30
  Mux : Mux  Inputs=3
  Outbound_Process_1 : InfiniteServer  ServiceTimeFrom=Signal port t  ServiceTime=(76.7)/30  StatNumberInBlock=on
      settings: OutputPortMap=o1
  Outbound_Process_2 : InfiniteServer  ServiceTimeFrom=Signal port t  ServiceTime=(76.7)/30  StatNumberInBlock=on
      settings: OutputPortMap=o1
  Outbound_Release_1 : SingleServer  ServiceTime=0  StatNumberInBlock=on
      settings: OutputPortMap=o1
  Outbound_Release_2 : SingleServer  ServiceTime=0  StatNumberInBlock=on
      settings: OutputPortMap=o1
  Sum{,1..2,4} (4 alike) : Sum  Inputs=|++
  Sum3 : Sum  Inputs=|++++
  TC_Status : simeventslib/SimEvents Sinks/Discrete Event Signal to Workspace  VariableName=Transportation_Channel_37_Status  SaveFormat=Structure With Time  isMonitorOnly=off  isRecordIC=off
  Timed to Event Signal : TimedToEventSignal
  TravelTime : Constant  Value=58.0035/30
  IN_Shipment_1 : PMIOPort  Port=1  Side=Left
  OUT_Shipment_1 : PMIOPort  Port=2  Side=Right
  IN_Resource_1 : PMIOPort  Port=3  Side=Left
  OUT_Resource_1 : PMIOPort  Port=4  Side=Right
  IN_Shipment_2 : PMIOPort  Port=5  Side=Left
  OUT_Shipment_2 : PMIOPort  Port=6  Side=Right
  IN_Resource_2 : PMIOPort  Port=7  Side=Left
  OUT_Resource_2 : PMIOPort  Port=8  Side=Right
  tag scope: Transportation_Channel_37_Status=global
  wires:
  Sum4/1 -> Mux/3
  Inbound_Process_2/1 -> Sum4/2
  Inbound_Process_1/1 -> Sum4/1
  Inbound_Process_2/2 -> Sum3/4
  Outbound_Process_2/1 -> Sum3/3
  Inbound_Process_1/2 -> Sum3/2
  Outbound_Process_1/1 -> Sum3/1
  Sum3/1 -> Mux/2
  Sum/1 -> Mux/1
  Mux/1 -> TC_Status/1, [Transportation_Channel_37_Status]
  Inbound_Release_2/1 -> Sum2/2
  Outbound_Release_1/1 -> Sum2/1
  Sum2/1 -> Enabled Gate/1
  Inbound_Release_1/1 -> Sum1/1
  Outbound_Release_2/1 -> Sum1/2
  Sum1/1 -> Enabled Gate1/1
  Timed to Event Signal/1 -> Infinite Server/1, Inbound_Process_2/1, Inbound_Process_1/1, Infinite Server1/1, Outbound_Process_2/1, Outbound_Process_1/1
  TravelTime/1 -> Timed to Event Signal/1
  FIFO Queue/1 -> Sum/1
  FIFO Queue1/1 -> Sum/2
  connections:
  Inbound_Process_1/RConn1 -- OUT_Resource_1/RConn1
  Outbound_Process_1/RConn1 -- Inbound_Release_1/LConn1
  Inbound_Release_1/RConn1 -- Inbound_Process_1/LConn1
  Outbound_Release_1/RConn1 -- Outbound_Process_1/LConn1
  Inbound_Process_2/RConn1 -- OUT_Resource_2/RConn1
  Inbound_Release_2/RConn1 -- Inbound_Process_2/LConn1
  Outbound_Process_2/RConn1 -- Inbound_Release_2/LConn1
  Outbound_Release_2/RConn1 -- Outbound_Process_2/LConn1
  IN_Resource_2/RConn1 -- Outbound_Release_2/LConn1
  Infinite Server1/RConn1 -- OUT_Shipment_1/RConn1
  Enabled Gate/RConn1 -- Infinite Server1/LConn1
  Infinite Server/LConn1 -- Enabled Gate1/RConn1
  OUT_Shipment_2/RConn1 -- Infinite Server/RConn1
  IN_Resource_1/RConn1 -- Outbound_Release_1/LConn1
  IN_Shipment_2/RConn1 -- FIFO Queue1/LConn1
  IN_Shipment_1/RConn1 -- FIFO Queue/LConn1
  Enabled Gate1/LConn1 -- FIFO Queue1/RConn1
  FIFO Queue/RConn1 -- Enabled Gate/LConn1

== system Distribution_v2/Transportation_Channel_38 ==
  note: RESOURCE1 OUTBOUND
      | RESOURCE2 INBOUND
  note: RESOURCE1 INBOUND
      | RESOURCE2 OUTBOUND
  Enabled Gate : EnabledGate
  Enabled Gate1 : EnabledGate
  FIFO Queue : FIFOQueue  Capacity=inf  StatNumberInBlock=on
      settings: OutputPortMap=o1
  FIFO Queue1 : FIFOQueue  Capacity=inf  StatNumberInBlock=on
      settings: OutputPortMap=o1
  Inbound_Process_1 : InfiniteServer  ServiceTimeFrom=Signal port t  ServiceTime=(76.7)/30  StatNumberDeparted=on  StatNumberInBlock=on
      settings: OutputPortMap=o0,o1
  Inbound_Process_2 : InfiniteServer  ServiceTimeFrom=Signal port t  ServiceTime=(76.7)/30  StatNumberDeparted=on  StatNumberInBlock=on
      settings: OutputPortMap=o0,o1
  Inbound_Release_1 : SingleServer  ServiceTime=0  StatNumberInBlock=on
      settings: OutputPortMap=o1
  Inbound_Release_2 : SingleServer  ServiceTime=0  StatNumberInBlock=on
      settings: OutputPortMap=o1
  Infinite Server : InfiniteServer  ServiceTimeFrom=Signal port t  ServiceTime=(76.7)/30
  Infinite Server1 : InfiniteServer  ServiceTimeFrom=Signal port t  ServiceTime=(76.7)/30
  Mux : Mux  Inputs=3
  Outbound_Process_1 : InfiniteServer  ServiceTimeFrom=Signal port t  ServiceTime=(76.7)/30  StatNumberInBlock=on
      settings: OutputPortMap=o1
  Outbound_Process_2 : InfiniteServer  ServiceTimeFrom=Signal port t  ServiceTime=(76.7)/30  StatNumberInBlock=on
      settings: OutputPortMap=o1
  Outbound_Release_1 : SingleServer  ServiceTime=0  StatNumberInBlock=on
      settings: OutputPortMap=o1
  Outbound_Release_2 : SingleServer  ServiceTime=0  StatNumberInBlock=on
      settings: OutputPortMap=o1
  Sum{,1..2,4} (4 alike) : Sum  Inputs=|++
  Sum3 : Sum  Inputs=|++++
  TC_Status : simeventslib/SimEvents Sinks/Discrete Event Signal to Workspace  VariableName=Transportation_Channel_38_Status  SaveFormat=Structure With Time  isMonitorOnly=off  isRecordIC=off
  Timed to Event Signal : TimedToEventSignal
  TravelTime : Constant  Value=86.1455/30
  IN_Shipment_1 : PMIOPort  Port=1  Side=Left
  OUT_Shipment_1 : PMIOPort  Port=2  Side=Right
  IN_Resource_1 : PMIOPort  Port=3  Side=Left
  OUT_Resource_1 : PMIOPort  Port=4  Side=Right
  IN_Shipment_2 : PMIOPort  Port=5  Side=Left
  OUT_Shipment_2 : PMIOPort  Port=6  Side=Right
  IN_Resource_2 : PMIOPort  Port=7  Side=Left
  OUT_Resource_2 : PMIOPort  Port=8  Side=Right
  tag scope: Transportation_Channel_38_Status=global
  wires:
  Sum4/1 -> Mux/3
  Inbound_Process_2/1 -> Sum4/2
  Inbound_Process_1/1 -> Sum4/1
  Inbound_Process_2/2 -> Sum3/4
  Outbound_Process_2/1 -> Sum3/3
  Inbound_Process_1/2 -> Sum3/2
  Outbound_Process_1/1 -> Sum3/1
  Sum3/1 -> Mux/2
  Sum/1 -> Mux/1
  Mux/1 -> TC_Status/1, [Transportation_Channel_38_Status]
  Inbound_Release_2/1 -> Sum2/2
  Outbound_Release_1/1 -> Sum2/1
  Sum2/1 -> Enabled Gate/1
  Inbound_Release_1/1 -> Sum1/1
  Outbound_Release_2/1 -> Sum1/2
  Sum1/1 -> Enabled Gate1/1
  Timed to Event Signal/1 -> Infinite Server/1, Inbound_Process_2/1, Inbound_Process_1/1, Infinite Server1/1, Outbound_Process_2/1, Outbound_Process_1/1
  TravelTime/1 -> Timed to Event Signal/1
  FIFO Queue/1 -> Sum/1
  FIFO Queue1/1 -> Sum/2
  connections:
  Inbound_Process_1/RConn1 -- OUT_Resource_1/RConn1
  Outbound_Process_1/RConn1 -- Inbound_Release_1/LConn1
  Inbound_Release_1/RConn1 -- Inbound_Process_1/LConn1
  Outbound_Release_1/RConn1 -- Outbound_Process_1/LConn1
  Inbound_Process_2/RConn1 -- OUT_Resource_2/RConn1
  Inbound_Release_2/RConn1 -- Inbound_Process_2/LConn1
  Outbound_Process_2/RConn1 -- Inbound_Release_2/LConn1
  Outbound_Release_2/RConn1 -- Outbound_Process_2/LConn1
  IN_Resource_2/RConn1 -- Outbound_Release_2/LConn1
  Infinite Server1/RConn1 -- OUT_Shipment_1/RConn1
  Enabled Gate/RConn1 -- Infinite Server1/LConn1
  Infinite Server/LConn1 -- Enabled Gate1/RConn1
  OUT_Shipment_2/RConn1 -- Infinite Server/RConn1
  IN_Resource_1/RConn1 -- Outbound_Release_1/LConn1
  IN_Shipment_2/RConn1 -- FIFO Queue1/LConn1
  IN_Shipment_1/RConn1 -- FIFO Queue/LConn1
  Enabled Gate1/LConn1 -- FIFO Queue1/RConn1
  FIFO Queue/RConn1 -- Enabled Gate/LConn1

== system Distribution_v2/Transportation_Channel_39 ==
  note: RESOURCE1 OUTBOUND
      | RESOURCE2 INBOUND
  note: RESOURCE1 INBOUND
      | RESOURCE2 OUTBOUND
  Enabled Gate : EnabledGate
  Enabled Gate1 : EnabledGate
  FIFO Queue : FIFOQueue  Capacity=inf  StatNumberInBlock=on
      settings: OutputPortMap=o1
  FIFO Queue1 : FIFOQueue  Capacity=inf  StatNumberInBlock=on
      settings: OutputPortMap=o1
  Inbound_Process_1 : InfiniteServer  ServiceTimeFrom=Signal port t  ServiceTime=(76.7)/30  StatNumberDeparted=on  StatNumberInBlock=on
      settings: OutputPortMap=o0,o1
  Inbound_Process_2 : InfiniteServer  ServiceTimeFrom=Signal port t  ServiceTime=(76.7)/30  StatNumberDeparted=on  StatNumberInBlock=on
      settings: OutputPortMap=o0,o1
  Inbound_Release_1 : SingleServer  ServiceTime=0  StatNumberInBlock=on
      settings: OutputPortMap=o1
  Inbound_Release_2 : SingleServer  ServiceTime=0  StatNumberInBlock=on
      settings: OutputPortMap=o1
  Infinite Server : InfiniteServer  ServiceTimeFrom=Signal port t  ServiceTime=(76.7)/30
  Infinite Server1 : InfiniteServer  ServiceTimeFrom=Signal port t  ServiceTime=(76.7)/30
  Mux : Mux  Inputs=3
  Outbound_Process_1 : InfiniteServer  ServiceTimeFrom=Signal port t  ServiceTime=(76.7)/30  StatNumberInBlock=on
      settings: OutputPortMap=o1
  Outbound_Process_2 : InfiniteServer  ServiceTimeFrom=Signal port t  ServiceTime=(76.7)/30  StatNumberInBlock=on
      settings: OutputPortMap=o1
  Outbound_Release_1 : SingleServer  ServiceTime=0  StatNumberInBlock=on
      settings: OutputPortMap=o1
  Outbound_Release_2 : SingleServer  ServiceTime=0  StatNumberInBlock=on
      settings: OutputPortMap=o1
  Sum{,1..2,4} (4 alike) : Sum  Inputs=|++
  Sum3 : Sum  Inputs=|++++
  TC_Status : simeventslib/SimEvents Sinks/Discrete Event Signal to Workspace  VariableName=Transportation_Channel_39_Status  SaveFormat=Structure With Time  isMonitorOnly=off  isRecordIC=off
  Timed to Event Signal : TimedToEventSignal
  TravelTime : Constant  Value=28.6443/30
  IN_Shipment_1 : PMIOPort  Port=1  Side=Left
  OUT_Shipment_1 : PMIOPort  Port=2  Side=Right
  IN_Resource_1 : PMIOPort  Port=3  Side=Left
  OUT_Resource_1 : PMIOPort  Port=4  Side=Right
  IN_Shipment_2 : PMIOPort  Port=5  Side=Left
  OUT_Shipment_2 : PMIOPort  Port=6  Side=Right
  IN_Resource_2 : PMIOPort  Port=7  Side=Left
  OUT_Resource_2 : PMIOPort  Port=8  Side=Right
  tag scope: Transportation_Channel_39_Status=global
  wires:
  Sum4/1 -> Mux/3
  Inbound_Process_2/1 -> Sum4/2
  Inbound_Process_1/1 -> Sum4/1
  Inbound_Process_2/2 -> Sum3/4
  Outbound_Process_2/1 -> Sum3/3
  Inbound_Process_1/2 -> Sum3/2
  Outbound_Process_1/1 -> Sum3/1
  Sum3/1 -> Mux/2
  Sum/1 -> Mux/1
  Mux/1 -> TC_Status/1, [Transportation_Channel_39_Status]
  Inbound_Release_2/1 -> Sum2/2
  Outbound_Release_1/1 -> Sum2/1
  Sum2/1 -> Enabled Gate/1
  Inbound_Release_1/1 -> Sum1/1
  Outbound_Release_2/1 -> Sum1/2
  Sum1/1 -> Enabled Gate1/1
  Timed to Event Signal/1 -> Infinite Server/1, Inbound_Process_2/1, Inbound_Process_1/1, Infinite Server1/1, Outbound_Process_2/1, Outbound_Process_1/1
  TravelTime/1 -> Timed to Event Signal/1
  FIFO Queue/1 -> Sum/1
  FIFO Queue1/1 -> Sum/2
  connections:
  Inbound_Process_1/RConn1 -- OUT_Resource_1/RConn1
  Outbound_Process_1/RConn1 -- Inbound_Release_1/LConn1
  Inbound_Release_1/RConn1 -- Inbound_Process_1/LConn1
  Outbound_Release_1/RConn1 -- Outbound_Process_1/LConn1
  Inbound_Process_2/RConn1 -- OUT_Resource_2/RConn1
  Inbound_Release_2/RConn1 -- Inbound_Process_2/LConn1
  Outbound_Process_2/RConn1 -- Inbound_Release_2/LConn1
  Outbound_Release_2/RConn1 -- Outbound_Process_2/LConn1
  IN_Resource_2/RConn1 -- Outbound_Release_2/LConn1
  Infinite Server1/RConn1 -- OUT_Shipment_1/RConn1
  Enabled Gate/RConn1 -- Infinite Server1/LConn1
  Infinite Server/LConn1 -- Enabled Gate1/RConn1
  OUT_Shipment_2/RConn1 -- Infinite Server/RConn1
  IN_Resource_1/RConn1 -- Outbound_Release_1/LConn1
  IN_Shipment_2/RConn1 -- FIFO Queue1/LConn1
  IN_Shipment_1/RConn1 -- FIFO Queue/LConn1
  Enabled Gate1/LConn1 -- FIFO Queue1/RConn1
  FIFO Queue/RConn1 -- Enabled Gate/LConn1

== system Distribution_v2/Transportation_Channel_40 ==
  note: RESOURCE1 OUTBOUND
      | RESOURCE2 INBOUND
  note: RESOURCE1 INBOUND
      | RESOURCE2 OUTBOUND
  Enabled Gate : EnabledGate
  Enabled Gate1 : EnabledGate
  FIFO Queue : FIFOQueue  Capacity=inf  StatNumberInBlock=on
      settings: OutputPortMap=o1
  FIFO Queue1 : FIFOQueue  Capacity=inf  StatNumberInBlock=on
      settings: OutputPortMap=o1
  Inbound_Process_1 : InfiniteServer  ServiceTimeFrom=Signal port t  ServiceTime=(76.7)/30  StatNumberDeparted=on  StatNumberInBlock=on
      settings: OutputPortMap=o0,o1
  Inbound_Process_2 : InfiniteServer  ServiceTimeFrom=Signal port t  ServiceTime=(76.7)/30  StatNumberDeparted=on  StatNumberInBlock=on
      settings: OutputPortMap=o0,o1
  Inbound_Release_1 : SingleServer  ServiceTime=0  StatNumberInBlock=on
      settings: OutputPortMap=o1
  Inbound_Release_2 : SingleServer  ServiceTime=0  StatNumberInBlock=on
      settings: OutputPortMap=o1
  Infinite Server : InfiniteServer  ServiceTimeFrom=Signal port t  ServiceTime=(76.7)/30
  Infinite Server1 : InfiniteServer  ServiceTimeFrom=Signal port t  ServiceTime=(76.7)/30
  Mux : Mux  Inputs=3
  Outbound_Process_1 : InfiniteServer  ServiceTimeFrom=Signal port t  ServiceTime=(76.7)/30  StatNumberInBlock=on
      settings: OutputPortMap=o1
  Outbound_Process_2 : InfiniteServer  ServiceTimeFrom=Signal port t  ServiceTime=(76.7)/30  StatNumberInBlock=on
      settings: OutputPortMap=o1
  Outbound_Release_1 : SingleServer  ServiceTime=0  StatNumberInBlock=on
      settings: OutputPortMap=o1
  Outbound_Release_2 : SingleServer  ServiceTime=0  StatNumberInBlock=on
      settings: OutputPortMap=o1
  Sum{,1..2,4} (4 alike) : Sum  Inputs=|++
  Sum3 : Sum  Inputs=|++++
  TC_Status : simeventslib/SimEvents Sinks/Discrete Event Signal to Workspace  VariableName=Transportation_Channel_40_Status  SaveFormat=Structure With Time  isMonitorOnly=off  isRecordIC=off
  Timed to Event Signal : TimedToEventSignal
  TravelTime : Constant  Value=30.3111/30
  IN_Shipment_1 : PMIOPort  Port=1  Side=Left
  OUT_Shipment_1 : PMIOPort  Port=2  Side=Right
  IN_Resource_1 : PMIOPort  Port=3  Side=Left
  OUT_Resource_1 : PMIOPort  Port=4  Side=Right
  IN_Shipment_2 : PMIOPort  Port=5  Side=Left
  OUT_Shipment_2 : PMIOPort  Port=6  Side=Right
  IN_Resource_2 : PMIOPort  Port=7  Side=Left
  OUT_Resource_2 : PMIOPort  Port=8  Side=Right
  tag scope: Transportation_Channel_40_Status=global
  wires:
  Sum4/1 -> Mux/3
  Inbound_Process_2/1 -> Sum4/2
  Inbound_Process_1/1 -> Sum4/1
  Inbound_Process_2/2 -> Sum3/4
  Outbound_Process_2/1 -> Sum3/3
  Inbound_Process_1/2 -> Sum3/2
  Outbound_Process_1/1 -> Sum3/1
  Sum3/1 -> Mux/2
  Sum/1 -> Mux/1
  Mux/1 -> TC_Status/1, [Transportation_Channel_40_Status]
  Inbound_Release_2/1 -> Sum2/2
  Outbound_Release_1/1 -> Sum2/1
  Sum2/1 -> Enabled Gate/1
  Inbound_Release_1/1 -> Sum1/1
  Outbound_Release_2/1 -> Sum1/2
  Sum1/1 -> Enabled Gate1/1
  Timed to Event Signal/1 -> Infinite Server/1, Inbound_Process_2/1, Inbound_Process_1/1, Infinite Server1/1, Outbound_Process_2/1, Outbound_Process_1/1
  TravelTime/1 -> Timed to Event Signal/1
  FIFO Queue/1 -> Sum/1
  FIFO Queue1/1 -> Sum/2
  connections:
  Inbound_Process_1/RConn1 -- OUT_Resource_1/RConn1
  Outbound_Process_1/RConn1 -- Inbound_Release_1/LConn1
  Inbound_Release_1/RConn1 -- Inbound_Process_1/LConn1
  Outbound_Release_1/RConn1 -- Outbound_Process_1/LConn1
  Inbound_Process_2/RConn1 -- OUT_Resource_2/RConn1
  Inbound_Release_2/RConn1 -- Inbound_Process_2/LConn1
  Outbound_Process_2/RConn1 -- Inbound_Release_2/LConn1
  Outbound_Release_2/RConn1 -- Outbound_Process_2/LConn1
  IN_Resource_2/RConn1 -- Outbound_Release_2/LConn1
  Infinite Server1/RConn1 -- OUT_Shipment_1/RConn1
  Enabled Gate/RConn1 -- Infinite Server1/LConn1
  Infinite Server/LConn1 -- Enabled Gate1/RConn1
  OUT_Shipment_2/RConn1 -- Infinite Server/RConn1
  IN_Resource_1/RConn1 -- Outbound_Release_1/LConn1
  IN_Shipment_2/RConn1 -- FIFO Queue1/LConn1
  IN_Shipment_1/RConn1 -- FIFO Queue/LConn1
  Enabled Gate1/LConn1 -- FIFO Queue1/RConn1
  FIFO Queue/RConn1 -- Enabled Gate/LConn1

== system Distribution_v2/Transportation_Channel_41 ==
  note: RESOURCE1 OUTBOUND
      | RESOURCE2 INBOUND
  note: RESOURCE1 INBOUND
      | RESOURCE2 OUTBOUND
  Enabled Gate : EnabledGate
  Enabled Gate1 : EnabledGate
  FIFO Queue : FIFOQueue  Capacity=inf  StatNumberInBlock=on
      settings: OutputPortMap=o1
  FIFO Queue1 : FIFOQueue  Capacity=inf  StatNumberInBlock=on
      settings: OutputPortMap=o1
  Inbound_Process_1 : InfiniteServer  ServiceTimeFrom=Signal port t  ServiceTime=(76.7)/30  StatNumberDeparted=on  StatNumberInBlock=on
      settings: OutputPortMap=o0,o1
  Inbound_Process_2 : InfiniteServer  ServiceTimeFrom=Signal port t  ServiceTime=(76.7)/30  StatNumberDeparted=on  StatNumberInBlock=on
      settings: OutputPortMap=o0,o1
  Inbound_Release_1 : SingleServer  ServiceTime=0  StatNumberInBlock=on
      settings: OutputPortMap=o1
  Inbound_Release_2 : SingleServer  ServiceTime=0  StatNumberInBlock=on
      settings: OutputPortMap=o1
  Infinite Server : InfiniteServer  ServiceTimeFrom=Signal port t  ServiceTime=(76.7)/30
  Infinite Server1 : InfiniteServer  ServiceTimeFrom=Signal port t  ServiceTime=(76.7)/30
  Mux : Mux  Inputs=3
  Outbound_Process_1 : InfiniteServer  ServiceTimeFrom=Signal port t  ServiceTime=(76.7)/30  StatNumberInBlock=on
      settings: OutputPortMap=o1
  Outbound_Process_2 : InfiniteServer  ServiceTimeFrom=Signal port t  ServiceTime=(76.7)/30  StatNumberInBlock=on
      settings: OutputPortMap=o1
  Outbound_Release_1 : SingleServer  ServiceTime=0  StatNumberInBlock=on
      settings: OutputPortMap=o1
  Outbound_Release_2 : SingleServer  ServiceTime=0  StatNumberInBlock=on
      settings: OutputPortMap=o1
  Sum{,1..2,4} (4 alike) : Sum  Inputs=|++
  Sum3 : Sum  Inputs=|++++
  TC_Status : simeventslib/SimEvents Sinks/Discrete Event Signal to Workspace  VariableName=Transportation_Channel_41_Status  SaveFormat=Structure With Time  isMonitorOnly=off  isRecordIC=off
  Timed to Event Signal : TimedToEventSignal
  TravelTime : Constant  Value=28.4699/30
  IN_Shipment_1 : PMIOPort  Port=1  Side=Left
  OUT_Shipment_1 : PMIOPort  Port=2  Side=Right
  IN_Resource_1 : PMIOPort  Port=3  Side=Left
  OUT_Resource_1 : PMIOPort  Port=4  Side=Right
  IN_Shipment_2 : PMIOPort  Port=5  Side=Left
  OUT_Shipment_2 : PMIOPort  Port=6  Side=Right
  IN_Resource_2 : PMIOPort  Port=7  Side=Left
  OUT_Resource_2 : PMIOPort  Port=8  Side=Right
  tag scope: Transportation_Channel_41_Status=global
  wires:
  Sum4/1 -> Mux/3
  Inbound_Process_2/1 -> Sum4/2
  Inbound_Process_1/1 -> Sum4/1
  Inbound_Process_2/2 -> Sum3/4
  Outbound_Process_2/1 -> Sum3/3
  Inbound_Process_1/2 -> Sum3/2
  Outbound_Process_1/1 -> Sum3/1
  Sum3/1 -> Mux/2
  Sum/1 -> Mux/1
  Mux/1 -> TC_Status/1, [Transportation_Channel_41_Status]
  Inbound_Release_2/1 -> Sum2/2
  Outbound_Release_1/1 -> Sum2/1
  Sum2/1 -> Enabled Gate/1
  Inbound_Release_1/1 -> Sum1/1
  Outbound_Release_2/1 -> Sum1/2
  Sum1/1 -> Enabled Gate1/1
  Timed to Event Signal/1 -> Infinite Server/1, Inbound_Process_2/1, Inbound_Process_1/1, Infinite Server1/1, Outbound_Process_2/1, Outbound_Process_1/1
  TravelTime/1 -> Timed to Event Signal/1
  FIFO Queue/1 -> Sum/1
  FIFO Queue1/1 -> Sum/2
  connections:
  Inbound_Process_1/RConn1 -- OUT_Resource_1/RConn1
  Outbound_Process_1/RConn1 -- Inbound_Release_1/LConn1
  Inbound_Release_1/RConn1 -- Inbound_Process_1/LConn1
  Outbound_Release_1/RConn1 -- Outbound_Process_1/LConn1
  Inbound_Process_2/RConn1 -- OUT_Resource_2/RConn1
  Inbound_Release_2/RConn1 -- Inbound_Process_2/LConn1
  Outbound_Process_2/RConn1 -- Inbound_Release_2/LConn1
  Outbound_Release_2/RConn1 -- Outbound_Process_2/LConn1
  IN_Resource_2/RConn1 -- Outbound_Release_2/LConn1
  Infinite Server1/RConn1 -- OUT_Shipment_1/RConn1
  Enabled Gate/RConn1 -- Infinite Server1/LConn1
  Infinite Server/LConn1 -- Enabled Gate1/RConn1
  OUT_Shipment_2/RConn1 -- Infinite Server/RConn1
  IN_Resource_1/RConn1 -- Outbound_Release_1/LConn1
  IN_Shipment_2/RConn1 -- FIFO Queue1/LConn1
  IN_Shipment_1/RConn1 -- FIFO Queue/LConn1
  Enabled Gate1/LConn1 -- FIFO Queue1/RConn1
  FIFO Queue/RConn1 -- Enabled Gate/LConn1
